simulink model "CarQuarterHorz"  (R2018b)
settings: Solver=VariableStepAuto  StartTime=0.0  StopTime=10.0  RelTol=1e-3
settings Model: Creator=reece  LastModifiedBy=reece

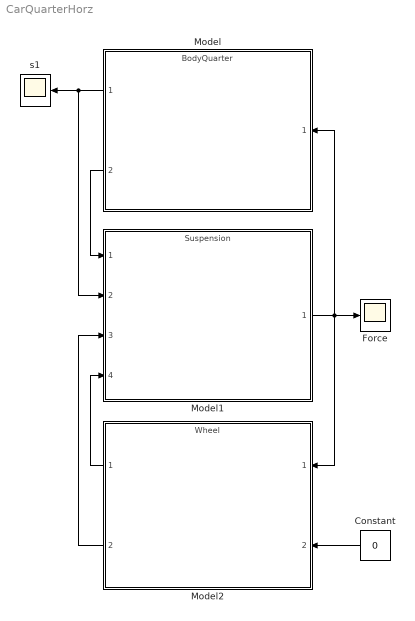
== system CarQuarterHorz ==
  Constant : Constant  Value=0
  Force : Scope
  Model : ModelReference  ModelNameDialog=BodyQuarter.slx  SimulationMode=Normal  ModelReferenceVersion=1.12
  Model1 : ModelReference  ModelNameDialog=Suspension.slx  SimulationMode=Normal  ModelReferenceVersion=1.7
  Model2 : ModelReference  ModelNameDialog=Wheel.slx  SimulationMode=Normal  ModelReferenceVersion=1.11
  s1 : Scope
  wires:
  Constant/1 -> Model2/2
  Model1/1 -> Force/1, Model/1, Model2/1
  Model2/2 -> Model1/3
  Model2/1 -> Model1/4
  Model/2 -> Model1/1
  Model/1 -> Model1/2, s1/1
